simulink model "AlgoritmiNewtonGradiente"  (R2021b)
settings: Solver=VariableStepAuto  StartTime=0.0  StopTime=3  RelTol=1e-3
settings Model: Creator=sugam  LastModifiedBy=sugam

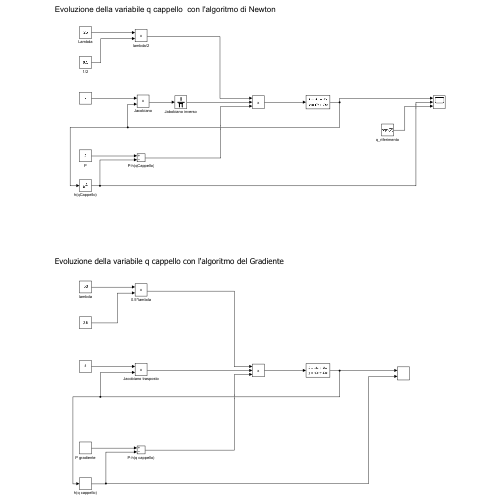
[thumbnail: Simulink's stored preview of the top-level diagram]
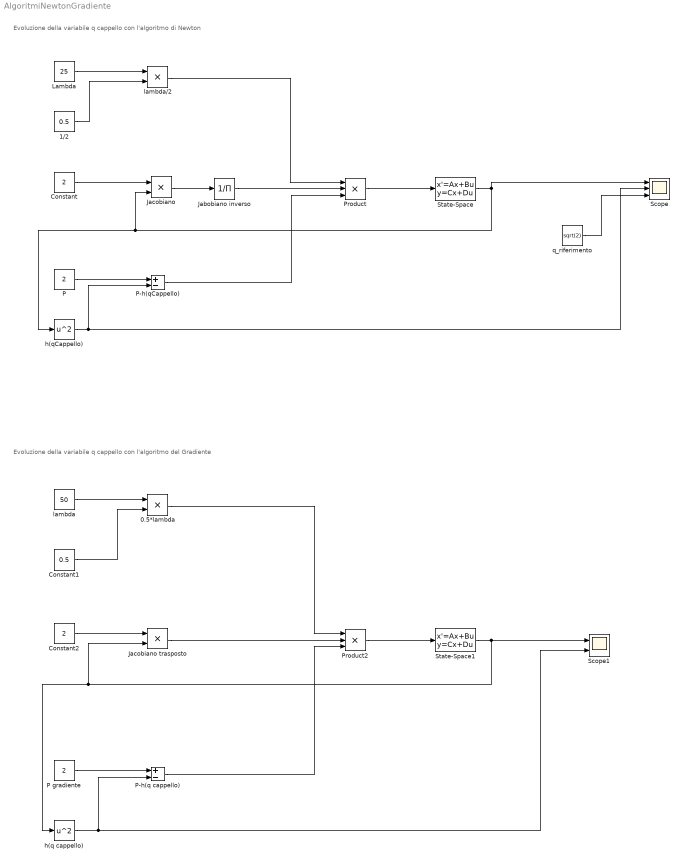
== system AlgoritmiNewtonGradiente ==
  note: Evoluzione della variabile q cappello con l'algoritmo del Gradiente
  note: Evoluzione della variabile q cappello con l'algoritmo di Newton
  0.5*lambda : Product
  1/2 : Constant  Value=0.5
  Constant : Constant  Value=2
  Constant1 : Constant  Value=0.5
  Constant2 : Constant  Value=2
  Jabobiano inverso : Product  Inputs=/  CollapseMode=Specified dimension
  Jacobiano : Product
  Jacobiano trasposto : Product
  Lambda : Constant  Value=25
  P : Constant  Value=2
  P gradiente : Constant  Value=2
  P-h(q cappello) : Sum  Inputs=+-
  P-h(qCappello) : Sum  Inputs=+-
  Product : Product  Inputs=3
  Product2 : Product  Inputs=3
  Scope : Scope  NumInputPorts=3
  Scope1 : Scope  NumInputPorts=2
  State-Space : StateSpace  A=0  D=0  InitialCondition=0.0001
  State-Space1 : StateSpace  A=0  D=0  InitialCondition=0.0001
  h(q cappello) : Math  Operator=square  SaturateOnIntegerOverflow=on
  h(qCappello) : Math  Operator=square  SaturateOnIntegerOverflow=on
  lambda : Constant  Value=50
  lambda/2 : Product
  q_riferimento : Constant  Value=sqrt(2)
  wires:
  Lambda/1 -> lambda/2/1
  1/2/1 -> lambda/2/2
  P/1 -> P-h(qCappello)/1
  h(qCappello)/1 -> Scope/2, P-h(qCappello)/2
  Constant/1 -> Jacobiano/1
  Jacobiano/1 -> Jabobiano inverso/1
  Product/1 -> State-Space/1
  lambda/2/1 -> Product/1
  Jabobiano inverso/1 -> Product/2
  P-h(qCappello)/1 -> Product/3
  State-Space/1 -> Scope/1, h(qCappello)/1, Jacobiano/2
  lambda/1 -> 0.5*lambda/1
  Constant1/1 -> 0.5*lambda/2
  P gradiente/1 -> P-h(q cappello)/1
  h(q cappello)/1 -> Scope1/2, P-h(q cappello)/2
  Constant2/1 -> Jacobiano trasposto/1
  0.5*lambda/1 -> Product2/1
  Jacobiano trasposto/1 -> Product2/2
  P-h(q cappello)/1 -> Product2/3
  Product2/1 -> State-Space1/1
  State-Space1/1 -> Scope1/1, h(q cappello)/1, Jacobiano trasposto/2
  q_riferimento/1 -> Scope/3
